simulink model "uav_full_control"  (R2023a)
settings: Solver=FixedStepAuto  StartTime=0.0  StopTime=20  FixedStep=1e-3
undefined symbols (not defined in the file or in its folder): b, c_1, c_2, c_3, c_4, c_5, c_6, c_7, c_8, c_psi, C_SMC, c_z, d, D_rot, D_transl, eps1, eps2, eps3, eps4, eta1, eta2, eta3, eta4, eulerlimit, g, J1, J2, J3, Jr, K, k1, k2, k3, K_lqr, k_phi, K_SMC, k_theta, L, m, Matrix_Force2angular_velocity, R
libraries: simulink x14, control_form_LagrangeSimplified x2, control_form_NL x2, control_form_NL_forces x2, control_form_LagrangeSimplified_forces x1
(part 1 of 2)
settings Model: Creator=Alex  LastModifiedBy=Alex

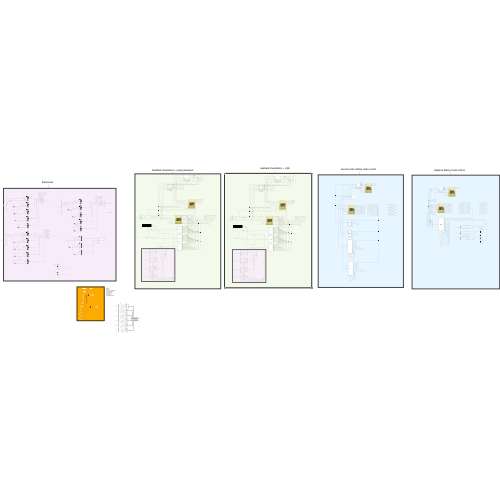
[thumbnail: Simulink's stored preview of the top-level diagram]
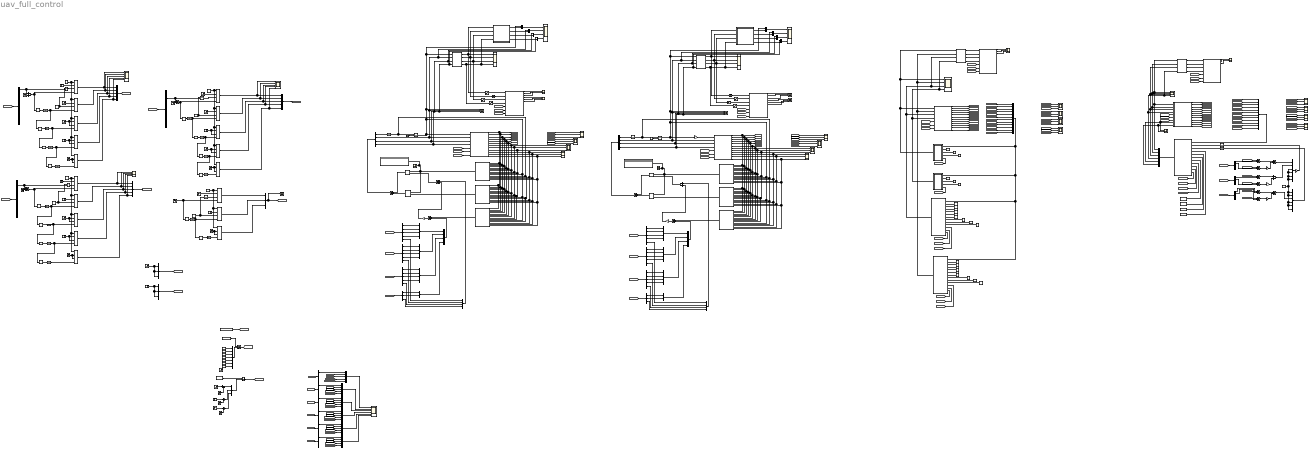
== system uav_full_control ==
  note: enables:
      | - gravity
      | - euler angles saturation
      | - gyroscopic effects
      | - ground effects
      | - drag force
      | - drag torques
      | - wind (translational)
  note: Feedback linearization + LQR
  note: 1 - step
      | 2 - ramp
      | 3 - else
  note: Feedback linearization + pole placement
  note: Adaptive Sliding mode control
  note: Second order sliding mode control
  note: References
  Add{,1,3..4,6..11} (10 alike) : Sum  Inputs=+-
  Add{2,5,12..17} (8 alike) : Sum
  Bus Creator{,1..5} (6 alike) : BusCreator  Inputs=5
  CNL_AngPos{,1..3} (4 alike) : Scope  NumInputPorts=3
  CNL_AngVel{,1..3} (4 alike) : Scope  NumInputPorts=3
  CNL_LinPos{,1..3} (4 alike) : Scope  NumInputPorts=3
  CNL_LinVel{,1..3} (4 alike) : Scope  NumInputPorts=3
  Constant : Constant  Value=K_SMC
  Constant11 : Constant  Value=k_phi
  Constant12 : Constant  Value=k_theta
  Constant13 : Constant  Value=C_SMC
  Constant14 : Constant  Value=0
  Constant15 : Constant  Value=eta1
  Constant16 : Constant  Value=c_z
  Constant17 : Constant  Value=eps3
  Constant20 : Constant  Value=eta3
  Constant21 : Constant  Value=eps4
  Constant22 : Constant  Value=eta4
  Constant23 : Constant  Value=c_5
  Constant24 : Constant  Value=c_6
  Constant25 : Constant  Value=c_7
  Constant26 : Constant  Value=c_8
  Constant29 : Constant  Value=eps1
  Constant3 : Constant  Value=2
  Constant30 : Constant  Value=eta1
  Constant31 : Constant  Value=c_z
  Constant32 : Constant  Value=eps1
  Constant33 : Constant  Value=eta1
  Constant34 : Constant  Value=c_z
  Constant35 : Constant  Value=eps1
  Constant36 : Constant  Value=eta2
  Constant37 : Constant  Value=c_psi
  Constant38 : Constant  Value=eps2
  Constant39 : Constant  Value=c_1
  Constant40 : Constant  Value=c_2
  Constant41 : Constant  Value=c_3
  Constant42 : Constant  Value=c_4
  Constant47 : Constant  Value=[1 0 0 0 1 1 0]
  Constant48 : Constant  Value=[1 1 -5 0 0 0 0 0 0 0 0 0 ]
  Constant49 : Constant  Value=[1 0 0]
  Constant8 : Constant  Value=2
  Demux : Demux
  Demux{1..3,6..8,10..12,14..16} (12 alike) : Demux  Outputs=5
  Demux13 : Demux  Outputs=6
  Demux{4,9,17..19} (5 alike) : Demux  Outputs=3
  Demux20 : Demux  Outputs=12
  Demux21 : Demux  Outputs=12
  Demux22 : Demux  Outputs=12
  Demux5 : Demux
  Discrete Derivative{,1..13} (14 alike) : simulink/Discrete/Discrete Derivative  gainval=1.0  ICPrevScaledInput=0.0  OutMin=[]  OutMax=[]  OutDataType=fixdt(1, 16)  OutScaling=2^-10  DoSatur=off
  Display : Display
  Display1 : Display
  Force2AngularVelocity : Subsystem
  Force2AngularVelocity1 : Subsystem
  Force2AngularVelocity2 : Subsystem
  Force2AngularVelocity3 : Subsystem
  Gain : Gain  Gain=k1
  Gain1 : Gain  Gain=-K_lqr  Multiplication=Matrix(K*u)
  Gain2 : Gain  Gain=-K  Multiplication=Matrix(K*u)
  Gain3 : Gain  Gain=k2
  Gain4 : Gain  Gain=k3
  Gain5 : Gain  Gain=-1
  Gain6 : Gain
  Input_psi : Constant
  Input_x : Constant
  Input_y : Constant
  Input_z : Constant
  Integrator{,2,4..5} (4 alike) : Integrator
  Integrator{1,3,6..7,16} (5 alike) : Integrator  InitialConditionSource=external
  Integrator21 : Integrator  LimitOutput=on  UpperSaturationLimit=pi  LowerSaturationLimit=-pi
  MATLAB Function : MATLAB Function  TreatAsAtomicUnit=on
  MATLAB Function1 : MATLAB Function  TreatAsAtomicUnit=on
  MATLAB Function2 : MATLAB Function  TreatAsAtomicUnit=on
  MATLAB Function3 : MATLAB Function  TreatAsAtomicUnit=on
  MATLAB Function4 : MATLAB Function  TreatAsAtomicUnit=on
  MATLAB Function5 : MATLAB Function  TreatAsAtomicUnit=on
  MATLAB Function6 : MATLAB Function  TreatAsAtomicUnit=on
  Manual Switch : ManualSwitch  CurrentSetting=0
  Manual Switch1 : ManualSwitch  CurrentSetting=0
  Matrix Multiply : Product  Multiplication=Matrix(*)
  Matrix Multiply1 : Product  Multiplication=Matrix(*)
  Multiport Switch{,1..17} (18 alike) : MultiPortSwitch  SaturateOnIntegerOverflow=off  InputSameDT=off
  Mux : Mux  Inputs=5
  Mux1 : Mux  Inputs=5
  Mux{8,10..17,22} (10 alike) : Mux  Inputs=2
  Mux{2,4,6..7,9,18..21,23} (10 alike) : Mux
  Mux24 : Mux  Inputs=12
  Mux25 : Mux  Inputs=6
  Mux26 : Mux  Inputs=6
  Mux{3,27,29,31} (4 alike) : Mux  Inputs=3
  Mux28 : Mux  Inputs=12
  Mux30 : Mux  Inputs=7
  Mux5 : Mux  Inputs=5
  Product : Product  Multiplication=Matrix(*)
  Product1 : Product  Multiplication=Matrix(*)
  STEP0_{1..16} (16 alike) : Step  Time=0  After=0  SampleTime=0
  Saturation{2..5,7..10} (8 alike) : Saturate  UpperLimit=1000  LowerLimit=0
  Scope : Scope
  Scope1 : Scope  NumInputPorts=5
  Scope10 : Scope
  Scope{5,8..9,11,14..17} (8 alike) : Scope  NumInputPorts=4
  Scope{6..7,12..13,18..19} (6 alike) : Scope  NumInputPorts=3
  Scope2 : Scope  NumInputPorts=5
  Scope20 : Scope  NumInputPorts=2
  Scope21 : Scope  NumInputPorts=6
  Scope3 : Scope  NumInputPorts=5
  Scope4 : Scope
  Sine Wave_psi : Sin  SampleTime=0
  Sine Wave_x : Sin  Frequency=0.5  SampleTime=0
  Sine Wave_y : Sin  Frequency=0.5  SampleTime=0
  Sine Wave_z : Sin  Frequency=0.5  SampleTime=0
  Slope_psi : Constant  Value=0.2
  Slope_x : Constant  Value=0.5
  Slope_y : Constant  Value=0.5
  Slope_z : Constant  Value=-1
  Step : Step  Time=25  SampleTime=0
  Step1 : Step  Time=25  SampleTime=0
  Step2 : Step  Time=35  SampleTime=0
  Step3 : Step  Time=50  SampleTime=0
  Step4 : Step  Time=60  SampleTime=0
  Step5 : Step  Time=75  SampleTime=0
  Step6 : Step  Time=85  SampleTime=0
  Step_psi : Step  Time=0  SampleTime=0
  Step_x : Step  Time=0  After=5  SampleTime=0
  Step_y : Step  Time=0  After=5  SampleTime=0
  Step_z : Step  Time=0  After=-7  SampleTime=0
  Subsystem1 : Subsystem
  Subsystem2 : Subsystem
  Sum : Sum  Inputs=|+-
  Sum1 : Sum  Inputs=|+-
  Sum2 : Sum  Inputs=|+-
  Transfer Fcn{,1..13} (14 alike) : TransferFcn  Denominator=[1 1]
  control_form_LagrangeSimplified : control_form_LagrangeSimplified/control_form_LagrangeSimplified  SystemSampleTime=-1  VariantActivationTime=update diagram  Latency=0  AutoFrameSizeCalculation=off
  control_form_LagrangeSimplified1 : control_form_LagrangeSimplified/control_form_LagrangeSimplified  SystemSampleTime=-1  VariantActivationTime=update diagram  Latency=0  AutoFrameSizeCalculation=off
  control_form_LagrangeSimplified_forces : control_form_LagrangeSimplified_forces/control_form_LagrangeSimplified_forces  SystemSampleTime=-1  VariantActivationTime=update diagram  Latency=0  AutoFrameSizeCalculation=off
  control_form_LagrangeSimplified_forces_augumented : Subsystem  AncestorBlock=control_form_LagrangeSimplified_forces/control_form_LagrangeSimplified_forces
  control_form_NL : control_form_NL/control_form_NL  SystemSampleTime=-1  VariantActivationTime=update diagram  Latency=0  AutoFrameSizeCalculation=off
  control_form_NL1 : control_form_NL/control_form_NL  SystemSampleTime=-1  VariantActivationTime=update diagram  Latency=0  AutoFrameSizeCalculation=off
  control_form_NL_forces : control_form_NL_forces/control_form_NL_forces  SystemSampleTime=-1  VariantActivationTime=update diagram  Latency=0  AutoFrameSizeCalculation=off
      settings: LibrarySourceBlock=control_form_NL_forces/control_form_NL
  control_form_NL_forces1 : control_form_NL_forces/control_form_NL_forces  SystemSampleTime=-1  VariantActivationTime=update diagram  Latency=0  AutoFrameSizeCalculation=off
      settings: LibrarySourceBlock=control_form_NL_forces/control_form_NL
  drag force : Constant
  drag torque : Constant
  euler_sat : Constant  Value=0
  gravity : Constant
  ground : Constant  Value=0
  gyro : Constant  Value=0
  u1 : MATLAB Function  TreatAsAtomicUnit=on
  u2 : MATLAB Function  TreatAsAtomicUnit=on
  u3 : MATLAB Function  TreatAsAtomicUnit=on
  u4 : MATLAB Function  TreatAsAtomicUnit=on
  wind : Constant  Value=0
  wires:
  control_form_NL_forces/3 -> MATLAB Function2/3(z), MATLAB Function1/3(z), MATLAB Function/3(z), [CNL_z_LQR]
  control_form_NL_forces/2 -> MATLAB Function2/2(y), MATLAB Function1/2(y), MATLAB Function/2(y), [CNL_y_LQR]
  control_form_NL_forces/1 -> MATLAB Function2/1(x), MATLAB Function1/1(x), MATLAB Function/1(x), [CNL_x_LQR]
  control_form_NL_forces/4 -> MATLAB Function2/4(phi), MATLAB Function1/4(phi), MATLAB Function/4(phi), [CNL_phi_LQR]
  control_form_NL_forces/5 -> MATLAB Function2/5(theta), MATLAB Function1/5(theta), MATLAB Function/5(theta), [CNL_theta_LQR]
  control_form_NL_forces/6 -> MATLAB Function2/6(psi), MATLAB Function1/6(psi), MATLAB Function/6(psi), [CNL_psi_LQR]
  [CNL_x_LQR] -> CNL_LinPos/1
  [CNL_y_LQR] -> CNL_LinPos/2
  [CNL_z_LQR] -> CNL_LinPos/3
  [CNL_phi_LQR] -> CNL_AngPos/1
  [CNL_theta_LQR] -> CNL_AngPos/2
  [CNL_psi_LQR] -> CNL_AngPos/3
  control_form_NL_forces/7 -> MATLAB Function2/7(xdot), MATLAB Function1/7(xdot), MATLAB Function/7(xdot), CNL_LinVel/1
  control_form_NL_forces/8 -> MATLAB Function2/8(ydot), MATLAB Function1/8(ydot), MATLAB Function/8(ydot), CNL_LinVel/2
  control_form_NL_forces/9 -> MATLAB Function/9(zdot), MATLAB Function2/9(zdot), MATLAB Function1/9(zdot), CNL_LinVel/3
  control_form_NL_forces/10 -> CNL_AngVel/1, MATLAB Function2/12(p), MATLAB Function1/12(p), MATLAB Function/12(p)
  control_form_NL_forces/11 -> CNL_AngVel/2, MATLAB Function2/13(q), MATLAB Function1/13(q), MATLAB Function/13(q)
  control_form_NL_forces/12 -> CNL_AngVel/3, MATLAB Function2/14(r), MATLAB Function1/14(r), MATLAB Function/14(r)
  Integrator/1 -> MATLAB Function/11(xi), MATLAB Function2/11(xi), MATLAB Function1/11(xi), Integrator1/1  "xi"
  Product/1 -> Add/2  "alpha"
  MATLAB Function1/1(b) -> Product/2
  MATLAB Function/1(delta_inv) -> Display/1, Scope/1, Matrix Multiply/1, Product/1  "beta"
  Matrix Multiply/1 -> Add/1
  Add1/1 -> Gain1/1  "z"
  Gain1/1 -> Add2/2  "v"
  Add/1 -> Demux/1
  Demux/1 -> Integrator/1  "u1_tilde"
  Integrator1/1 -> Gain6/1, MATLAB Function2/10(zeta), MATLAB Function1/10(zeta), MATLAB Function/10(zeta), Mux10/1, Force2AngularVelocity/1(u1), Scope5/1  "zeta"
  Step_x/1 -> Multiport Switch/2
  Mux/1 -> [xref]
  Constant3/1 -> Integrator1/2
  Mux1/1 -> [yref]
  Step_psi/1 -> Multiport Switch15/2
  Mux3/1 -> [psiref], Scope4/1
  MATLAB Function2/1(transf) -> Add1/1  "z"
  Mux4/1 -> Add1/2
  Input_x/1 -> Multiport Switch4/1, Multiport Switch3/1, Multiport Switch2/1, Multiport Switch1/1, Multiport Switch/1
  STEP0_1/1 -> Multiport Switch1/2
  STEP0_2/1 -> Multiport Switch2/3, Multiport Switch2/2
  STEP0_3/1 -> Multiport Switch3/3, Multiport Switch3/2
  STEP0_4/1 -> Multiport Switch4/3, Multiport Switch4/2
  Multiport Switch/1 -> Scope1/1, Mux/1
  Multiport Switch1/1 -> Scope1/2, Mux/2
  Multiport Switch2/1 -> Scope1/3, Mux/3
  Multiport Switch3/1 -> Scope1/4, Mux/4
  Multiport Switch4/1 -> Scope1/5, Mux/5
  Multiport Switch9/1 -> Scope2/5, Mux1/5
  Multiport Switch8/1 -> Scope2/4, Mux1/4
  Multiport Switch7/1 -> Scope2/3, Mux1/3
  Multiport Switch6/1 -> Scope2/2, Mux1/2
  Multiport Switch5/1 -> Scope2/1, Mux1/1
  STEP0_8/1 -> Multiport Switch9/2, Multiport Switch9/3
  STEP0_7/1 -> Multiport Switch8/2, Multiport Switch8/3
  STEP0_6/1 -> Multiport Switch7/2, Multiport Switch7/3
  STEP0_5/1 -> Multiport Switch6/2
  Input_y/1 -> Multiport Switch5/1, Multiport Switch6/1, Multiport Switch7/1, Multiport Switch8/1, Multiport Switch9/1
  Step_y/1 -> Multiport Switch5/2
  Step_z/1 -> Multiport Switch10/2
  Input_z/1 -> Multiport Switch14/1, Multiport Switch13/1, Multiport Switch12/1, Multiport Switch11/1, Multiport Switch10/1
  STEP0_9/1 -> Multiport Switch11/2
  STEP0_10/1 -> Multiport Switch12/3, Multiport Switch12/2
  STEP0_11/1 -> Multiport Switch13/3, Multiport Switch13/2
  STEP0_12/1 -> Multiport Switch14/3, Multiport Switch14/2
  Multiport Switch10/1 -> Scope3/1, Mux5/1
  Multiport Switch11/1 -> Scope3/2, Mux5/2
  Multiport Switch12/1 -> Scope3/3, Mux5/3
  Multiport Switch13/1 -> Scope3/4, Mux5/4
  Multiport Switch14/1 -> Mux5/5, Scope3/5
  Mux5/1 -> [zref]
  Input_psi/1 -> Multiport Switch17/1, Multiport Switch16/1, Multiport Switch15/1
  STEP0_13/1 -> Multiport Switch16/2
  STEP0_14/1 -> Multiport Switch17/3, Multiport Switch17/2
  Sine Wave_psi/1 -> Discrete Derivative/1, Multiport Switch15/4
  [xref] -> Demux1/1
  Demux1/1 -> Mux2/1
  Demux1/2 -> Mux2/2
  Demux1/3 -> Mux2/3
  Demux1/4 -> Mux2/4
  Mux2/1 -> Mux4/1
  Mux6/1 -> Mux4/2
  Demux2/4 -> Mux6/4
  Demux2/3 -> Mux6/3
  Demux2/2 -> Mux6/2
  Demux2/1 -> Mux6/1
  [yref] -> Demux2/1
  [zref] -> Demux3/1
  Demux3/1 -> Mux7/1
  Demux3/2 -> Mux7/2
  Demux3/3 -> Mux7/3
  Demux3/4 -> Mux7/4
  Mux7/1 -> Mux4/3
  [psiref] -> Demux4/1
  Demux4/1 -> Mux8/1
  Demux4/2 -> Mux8/2
  Mux8/1 -> Mux4/4
  Demux4/3 -> Mux9/4
  Demux3/5 -> Mux9/3
  Demux2/5 -> Mux9/2
  Demux1/5 -> Mux9/1
  Mux9/1 -> Add2/1
  Add2/1 -> Matrix Multiply/2
  control_form_NL/1 -> Scope6/1
  control_form_NL/2 -> Scope6/2
  control_form_NL/3 -> Scope6/3
  control_form_NL/4 -> Scope7/1
  control_form_NL/5 -> Scope7/2
  control_form_NL/6 -> Scope7/3
  Force2AngularVelocity/1(omega_f) -> Subsystem1/1(omega_f), Scope8/1, Saturation2/1  "lqr_front"
  Force2AngularVelocity/2(omega_b) -> Subsystem1/2(omega_b), Scope8/2, Saturation3/1  "lqr_back"
  Force2AngularVelocity/3(omega_l) -> Subsystem1/3(omega_l), Scope8/3, Saturation4/1  "lqr_left"
  Force2AngularVelocity/4(omega_r) -> Saturation5/1, Subsystem1/4(omega_r), Scope8/4  "lqr_right"
  Demux/4 -> control_form_NL_forces/4, Mux13/1, Force2AngularVelocity/4(u4), Scope5/4  "lqr_M3"
  Demux/3 -> control_form_NL_forces/3, Mux12/1, Force2AngularVelocity/3(u3), Scope5/3  "lqr_M2"
  Demux/2 -> control_form_NL_forces/2, Mux11/1, Force2AngularVelocity/2(u2), Scope5/2  "lqr_M1"
  Multiport Switch15/1 -> Mux3/1
  Multiport Switch16/1 -> Mux3/2
  Multiport Switch17/1 -> Mux3/3
  Subsystem1/1(Thrust) -> Mux10/2
  Subsystem1/2(M1) -> Mux11/2
  Subsystem1/3(M2) -> Mux12/2
  Subsystem1/4(M3) -> Mux13/2
  Mux13/1 -> Scope9/4
  Mux12/1 -> Scope9/3
  Mux11/1 -> Scope9/2
  Mux10/1 -> Scope9/1
  Saturation2/1 -> control_form_NL/1
  Saturation3/1 -> control_form_NL/2
  Saturation4/1 -> control_form_NL/3
  Saturation5/1 -> control_form_NL/4
  Mux14/1 -> Scope15/1
  [xref] -> Demux6/1
  Mux16/1 -> Scope15/3
  control_form_NL1/3 -> Scope12/3
  Mux15/1 -> Scope15/2
  Subsystem2/1(Thrust) -> Mux14/2
  Mux17/1 -> Scope15/4
  Demux5/3 -> control_form_NL_forces1/3, Mux16/1, Force2AngularVelocity1/3(u3), Scope11/3  "pp_M2"
  control_form_NL_forces1/4 -> MATLAB Function5/4(phi), MATLAB Function4/4(phi), MATLAB Function3/4(phi), [CNL_phi_PP]
  Subsystem2/2(M1) -> Mux15/2
  Integrator3/1 -> control_form_NL_forces1/1, MATLAB Function5/10(zeta), MATLAB Function4/10(zeta), MATLAB Function3/10(zeta), Mux14/1, Force2AngularVelocity1/1(u1), Scope11/1  "pp_F_thrust"
  Mux23/1 -> Add5/1
  control_form_NL_forces1/5 -> MATLAB Function5/5(theta), MATLAB Function4/5(theta), MATLAB Function3/5(theta), [CNL_theta_PP]
  Demux6/5 -> Mux23/1
  Mux22/1 -> Mux19/4
  Demux7/5 -> Mux23/2
  control_form_NL_forces1/12 -> CNL_AngVel1/3, MATLAB Function5/14(r), MATLAB Function4/14(r), MATLAB Function3/14(r)
  Demux5/4 -> control_form_NL_forces1/4, Mux17/1, Force2AngularVelocity1/4(u4), Scope11/4  "pp_M3"
  Demux6/1 -> Mux18/1
  Demux9/2 -> Mux22/2
  Mux19/1 -> Add4/2
  MATLAB Function4/1(b) -> Product1/2
  Force2AngularVelocity1/4(omega_r) -> Saturation10/1, Subsystem2/4(omega_r), Scope14/4  "pp_right"
  Constant8/1 -> Integrator3/2
  Demux7/2 -> Mux20/2
  Force2AngularVelocity1/3(omega_l) -> Subsystem2/3(omega_l), Scope14/3, Saturation9/1  "pp_left"
  Demux7/3 -> Mux20/3
  control_form_NL1/6 -> Scope13/3
  Demux8/4 -> Mux21/4
  Demux8/5 -> Mux23/3
  Demux9/1 -> Mux22/1
  Mux21/1 -> Mux19/3
  Add5/1 -> Matrix Multiply1/2
  Demux7/1 -> Mux20/1
  Demux9/3 -> Mux23/4
  control_form_NL1/1 -> Scope12/1
  Demux6/3 -> Mux18/3
  control_form_NL1/4 -> Scope13/1
  [yref] -> Demux7/1
  Demux8/2 -> Mux21/2
  Demux8/3 -> Mux21/3
  Demux5/2 -> control_form_NL_forces1/2, Mux15/1, Force2AngularVelocity1/2(u2), Scope11/2  "pp_M1"
  Demux7/4 -> Mux20/4
  control_form_NL1/2 -> Scope12/2
  Demux6/2 -> Mux18/2
  [CNL_y_PP] -> CNL_LinPos1/2
  Mux20/1 -> Mux19/2
  Mux18/1 -> Mux19/1
  Demux6/4 -> Mux18/4
  control_form_NL1/5 -> Scope13/2
  control_form_NL_forces1/9 -> MATLAB Function3/9(zdot), MATLAB Function5/9(zdot), MATLAB Function4/9(zdot), CNL_LinVel1/3
  Force2AngularVelocity1/2(omega_b) -> Subsystem2/2(omega_b), Scope14/2, Saturation8/1  "pp_back"
  Matrix Multiply1/1 -> Add3/1
  MATLAB Function3/1(delta_inv) -> Display1/1, Scope10/1, Matrix Multiply1/1, Product1/1  "beta"
  Demux5/1 -> Integrator2/1  "u1_tilde"
  Add4/1 -> Gain2/1  "z"
  [zref] -> Demux8/1
  MATLAB Function5/1(transf) -> Add4/1  "z"
  control_form_NL_forces1/11 -> CNL_AngVel1/2, MATLAB Function5/13(q), MATLAB Function4/13(q), MATLAB Function3/13(q)
  Subsystem2/3(M2) -> Mux16/2
  Force2AngularVelocity1/1(omega_f) -> Subsystem2/1(omega_f), Scope14/1, Saturation7/1  "pp_front"
  control_form_NL_forces1/8 -> MATLAB Function5/8(ydot), MATLAB Function4/8(ydot), MATLAB Function3/8(ydot), CNL_LinVel1/2
  Gain2/1 -> Add5/2  "v"
  control_form_NL_forces1/2 -> MATLAB Function5/2(y), MATLAB Function4/2(y), MATLAB Function3/2(y), [CNL_y_PP]
  control_form_NL_forces1/3 -> MATLAB Function5/3(z), MATLAB Function4/3(z), MATLAB Function3/3(z), [CNL_z_PP]
  Integrator2/1 -> MATLAB Function3/11(xi), MATLAB Function5/11(xi), MATLAB Function4/11(xi), Integrator3/1  "xi"
  control_form_NL_forces1/7 -> MATLAB Function5/7(xdot), MATLAB Function4/7(xdot), MATLAB Function3/7(xdot), CNL_LinVel1/1
  Product1/1 -> Add3/2  "alpha"
  Subsystem2/4(M3) -> Mux17/2
  Add3/1 -> Demux5/1
  [CNL_phi_PP] -> CNL_AngPos1/1
  Demux8/1 -> Mux21/1
  [CNL_x_PP] -> CNL_LinPos1/1
  [psiref] -> Demux9/1
  [CNL_psi_PP] -> CNL_AngPos1/3
  control_form_NL_forces1/6 -> MATLAB Function5/6(psi), MATLAB Function4/6(psi), MATLAB Function3/6(psi), [CNL_psi_PP]
  control_form_NL_forces1/1 -> MATLAB Function5/1(x), MATLAB Function4/1(x), MATLAB Function3/1(x), [CNL_x_PP]
  [CNL_z_PP] -> CNL_LinPos1/3
  [CNL_theta_PP] -> CNL_AngPos1/2
  control_form_NL_forces1/10 -> CNL_AngVel1/1, MATLAB Function5/12(p), MATLAB Function4/12(p), MATLAB Function3/12(p)
  Saturation7/1 -> control_form_NL1/1
  Saturation8/1 -> control_form_NL1/2
  Saturation9/1 -> control_form_NL1/3
  Saturation10/1 -> control_form_NL1/4
  Add9/1 -> Gain3/1  "ey_dot"
  Add6/1 -> Add12/1  "ex"
  Integrator4/1 -> MATLAB Function6/2(v_hat)
  [CLS_z_ASMC] -> Mux24/3
  Add12/1 -> Mux25/1
  [yref] -> MATLAB Function6/9(yref)
  [CLS_xdot_ASMC] -> Add7/1
  Demux12/2 -> Add7/2
  Demux12/1 -> Add6/2
  Integrator5/1 -> MATLAB Function6/3(fr_hat)
  Demux10/1 -> Add10/2
  [zref] -> Demux10/1
  [psiref] -> MATLAB Function6/11(psiref)
  [xref] -> Demux12/1
  Demux11/1 -> Add8/2
  [CLS_psidot_ASMC] -> CNL_AngVel2/3
  Constant12/1 -> MATLAB Function6/5(k_theta)
  [CLS_psi_ASMC] -> CNL_AngPos2/3
  [CLS_zdot_ASMC] -> CNL_LinVel2/3
  [CLS_psi_ASMC] -> Mux24/6
  [CLS_theta_ASMC] -> Mux24/5
  control_form_LagrangeSimplified_forces_augumented/4(phi) -> [CLS_phi_ASMC]
  [CLS_phi_ASMC] -> Mux24/4
  Constant13/1 -> MATLAB Function6/4(C_SMC)
  [zref] -> MATLAB Function6/10(zref)
  [CLS_z_ASMC] -> CNL_LinPos2/3
  [CLS_zdot_ASMC] -> Mux24/9
  Constant/1 -> MATLAB Function6/7(K_SMC)
  [CLS_psidot_ASMC] -> Mux24/12
  [CLS_phi_ASMC] -> CNL_AngPos2/1
  [CLS_ydot_ASMC] -> Mux24/8
  [CLS_ydot_ASMC] -> CNL_LinVel2/2
  [CLS_y_ASMC] -> Mux24/2
  [CLS_phidot_ASMC] -> Mux24/10
  [CLS_xdot_ASMC] -> Mux24/7
  Mux24/1 -> MATLAB Function6/1(states)
  control_form_LagrangeSimplified_forces_augumented/2(y) -> [CLS_y_ASMC]
  [CLS_thetadot_ASMC] -> Mux24/11
  control_form_LagrangeSimplified_forces_augumented/5(theta) -> [CLS_theta_ASMC]
  control_form_LagrangeSimplified_forces_augumented/6(psi) -> [CLS_psi_ASMC]
  control_form_LagrangeSimplified_forces_augumented/3(z) -> [CLS_z_ASMC]
  control_form_LagrangeSimplified_forces_augumented/10(phidot) -> [CLS_phidot_ASMC]
  control_form_LagrangeSimplified_forces_augumented/7(xdot) -> [CLS_xdot_ASMC]
  [CLS_thetadot_ASMC] -> CNL_AngVel2/2
  [xref] -> MATLAB Function6/8(xref)
  Demux13/2 -> control_form_LagrangeSimplified_forces_augumented/2(M1), Force2AngularVelocity3/2(u2), Scope16/2  "ASMC_M1"
  control_form_LagrangeSimplified_forces_augumented/8(ydot) -> [CLS_ydot_ASMC]
  Demux13/4 -> control_form_LagrangeSimplified_forces_augumented/4(M3), Force2AngularVelocity3/4(u4), Scope16/4  "ASMC_M3"
  Demux13/5 -> Scope20/1, control_form_LagrangeSimplified_forces_augumented/8(u5)
  Demux13/3 -> Scope16/3, Force2AngularVelocity3/3(u3), control_form_LagrangeSimplified_forces_augumented/3(M2)  "ASMC_M2"
  [CLS_x_ASMC] -> CNL_LinPos2/1
  control_form_LagrangeSimplified_forces_augumented/1(x) -> [CLS_x_ASMC]
  control_form_LagrangeSimplified_forces_augumented/11(thetadot) -> [CLS_thetadot_ASMC]
  [CLS_x_ASMC] -> Add6/1
  Add8/1 -> Add13/1  "ey"
  Add10/1 -> Add14/1  "ez"
  Gain4/1 -> Add14/2
  Mux26/1 -> Integrator5/1
  Mux25/1 -> Gain5/1
  [CLS_phidot_ASMC] -> CNL_AngVel2/1
  Gain5/1 -> Integrator4/1
  Add11/1 -> Gain4/1  "ez_dot"
  [CLS_x_ASMC] -> Mux24/1
  [CLS_xdot_ASMC] -> CNL_LinVel2/1
  control_form_LagrangeSimplified_forces_augumented/12(psidot) -> [CLS_psidot_ASMC]
  Add13/1 -> Mux25/2
  Add7/1 -> Gain/1  "ex_dot"
  Demux10/2 -> Add11/2
  Demux11/2 -> Add9/2
  Add14/1 -> Mux26/3
  Demux13/1 -> Force2AngularVelocity3/1(u1), Scope16/1, control_form_LagrangeSimplified_forces_augumented/1(F_thrust)  "ASMC_F_Thrust"
  [CLS_y_ASMC] -> CNL_LinPos2/2
  [CLS_theta_ASMC] -> CNL_AngPos2/2
  [CLS_zdot_ASMC] -> Add11/1
  Constant14/1 -> Mux25/4, Mux25/3, Mux25/5, Mux25/6, Mux26/6, Mux26/5, Mux26/4, Mux26/2, Mux26/1
  Constant11/1 -> MATLAB Function6/6(k_phi)
  control_form_LagrangeSimplified_forces_augumented/9(zdot) -> [CLS_zdot_ASMC]
  Gain3/1 -> Add13/2
  Gain/1 -> Add12/2
  [CLS_z_ASMC] -> Add10/1
  [CLS_y_ASMC] -> Add8/1
  MATLAB Function6/1(u) -> Demux13/1
  [yref] -> Demux11/1
  [CLS_ydot_ASMC] -> Add9/1
  Demux13/6 -> Scope20/2, control_form_LagrangeSimplified_forces_augumented/9(u6)
  Constant32/1 -> u3/9(eps1)
  [thetaref] -> u3/13(thetaref)
  u2/1(u2) -> control_form_LagrangeSimplified_forces/2, Force2AngularVelocity2/2(u2), Scope17/2  "SMC2_M1"
  [CLS_phidot_2SMC] -> CNL_AngVel3/1
  u3/1(u3) -> control_form_LagrangeSimplified_forces/3, Force2AngularVelocity2/3(u3), Scope17/3  "SMC2_M2"
  Constant37/1 -> u4/2(c_psi)
  Constant21/1 -> u2/6(eps4)
  Constant23/1 -> u2/2(c_5)
  Constant34/1 -> u2/8(c_z)
  Constant33/1 -> u2/10(eta1)
  Constant35/1 -> u2/9(eps1)
  control_form_LagrangeSimplified_forces/7 -> [CLS_xdot_2SMC]
  Constant36/1 -> u4/4(eta2)
  Constant31/1 -> u3/8(c_z)
  control_form_LagrangeSimplified_forces/4 -> [CLS_phi_2SMC]
  Constant30/1 -> u3/10(eta1)
  u4/1(u4) -> control_form_LagrangeSimplified_forces/4, Force2AngularVelocity2/4(u4), Scope17/4  "SMC2_M3"
  Constant25/1 -> u2/4(c_7)
  [CLS_zdot_2SMC] -> CNL_LinVel3/3
  Constant42/1 -> u3/5(c_4)
  [CLS_x_2SMC] -> Mux28/1
  control_form_LagrangeSimplified_forces/11 -> [CLS_thetadot_2SMC]
  Constant22/1 -> u2/7(eta4)
  Constant39/1 -> u3/2(c_1)
  Constant26/1 -> u2/5(c_8)
  [CLS_z_2SMC] -> Mux28/3
  Constant24/1 -> u2/3(c_6)
  Constant16/1 -> u1/2(c_z)
  [yref] -> u2/12(yref)
  Constant41/1 -> u3/4(c_3)
  [CLS_psidot_2SMC] -> Mux28/12
  [CLS_xdot_2SMC] -> CNL_LinVel3/1
  [CLS_y_2SMC] -> CNL_LinPos3/2
  [zref] -> u1/5(zref)
  Constant38/1 -> u4/3(eps2)
  [CLS_thetadot_2SMC] -> CNL_AngVel3/2
  [zref] -> u3/11(zref)
  [zref] -> u2/11(zref)
  [xref] -> u3/12(xref)
  Mux28/1 -> u2/1(states), u3/1(states), u4/1(states), u1/1(states)
  Constant20/1 -> u3/7(eta3)
  [CLS_theta_2SMC] -> CNL_AngPos3/2
  [CLS_phidot_2SMC] -> Mux28/10
  Constant29/1 -> u1/3(eps1)
  [CLS_psi_2SMC] -> CNL_AngPos3/3
  control_form_LagrangeSimplified_forces/12 -> [CLS_psidot_2SMC]
  [CLS_ydot_2SMC] -> Mux28/8
  [CLS_theta_2SMC] -> Mux28/5
  control_form_LagrangeSimplified_forces/6 -> [CLS_psi_2SMC]
  [phiref] -> u2/13(phiref)
  [psiref] -> u4/5(psiref)
  [CLS_z_2SMC] -> CNL_LinPos3/3
  [CLS_zdot_2SMC] -> Mux28/9
  control_form_LagrangeSimplified_forces/5 -> [CLS_theta_2SMC]
  u1/1(u1) -> control_form_LagrangeSimplified_forces/1, Scope17/1, Force2AngularVelocity2/1(u1)  "SMC2_F_Thrust"
  control_form_LagrangeSimplified_forces/10 -> [CLS_phidot_2SMC]
  [CLS_thetadot_2SMC] -> Mux28/11
  [CLS_phi_2SMC] -> CNL_AngPos3/1
  control_form_LagrangeSimplified_forces/9 -> [CLS_zdot_2SMC]
  [CLS_psi_2SMC] -> Mux28/6
  Constant15/1 -> u1/4(eta1)
  [CLS_y_2SMC] -> Mux28/2
  control_form_LagrangeSimplified_forces/3 -> [CLS_z_2SMC]
  control_form_LagrangeSimplified_forces/2 -> [CLS_y_2SMC]
  [CLS_phi_2SMC] -> Mux28/4
  Constant17/1 -> u3/6(eps3)
  [CLS_ydot_2SMC] -> CNL_LinVel3/2
  [CLS_psidot_2SMC] -> CNL_AngVel3/3
  Constant40/1 -> u3/3(c_2)
  control_form_LagrangeSimplified_forces/8 -> [CLS_ydot_2SMC]
  [CLS_xdot_2SMC] -> Mux28/7
  control_form_LagrangeSimplified_forces/1 -> [CLS_x_2SMC]
  [CLS_x_2SMC] -> CNL_LinPos3/1
  Mux29/1 -> [phiref]
  STEP0_16/1 -> Mux29/1, Mux29/2, Mux29/3
  STEP0_15/1 -> Mux27/2, Mux27/3, Mux27/1
  Mux27/1 -> [thetaref]
  Force2AngularVelocity2/1(omega_f) -> control_form_LagrangeSimplified1/1  "SMC2_front"
  Force2AngularVelocity2/2(omega_b) -> control_form_LagrangeSimplified1/2  "SMC2_back"
  Force2AngularVelocity2/3(omega_l) -> control_form_LagrangeSimplified1/3  "SMC2_left"
  Force2AngularVelocity2/4(omega_r) -> control_form_LagrangeSimplified1/4  "SMC2_right"
  Force2AngularVelocity3/1(omega_f) -> control_form_LagrangeSimplified/1  "ASMC_front"
  Force2AngularVelocity3/2(omega_b) -> control_form_LagrangeSimplified/2  "ASMC_back"
  Force2AngularVelocity3/3(omega_l) -> control_form_LagrangeSimplified/3  "ASMC_left"
  Force2AngularVelocity3/4(omega_r) -> control_form_LagrangeSimplified/4  "ASMC_right"
  control_form_LagrangeSimplified1/1 -> Scope18/1
  control_form_LagrangeSimplified1/2 -> Scope18/2
  control_form_LagrangeSimplified1/3 -> Scope18/3
  control_form_LagrangeSimplified/1 -> Scope19/1
  control_form_LagrangeSimplified/2 -> Scope19/2
  control_form_LagrangeSimplified/3 -> Scope19/3
  Constant48/1 -> [initial_values]
  Manual Switch/1 -> [enables]
  Constant49/1 -> Manual Switch1/1
  [initial_values] -> control_form_NL1/5
  [enables] -> control_form_NL1/6
  [wind_power] -> control_form_NL1/7
  [initial_values] -> control_form_NL_forces1/5
  [enables] -> control_form_NL_forces1/6
  [wind_power] -> control_form_NL_forces1/7
  [initial_values] -> control_form_NL_forces/5
  [enables] -> control_form_NL_forces/6
  [wind_power] -> control_form_NL_forces/7
  [initial_values] -> control_form_NL/5
  [enables] -> control_form_NL/6
  [wind_power] -> control_form_NL/7
  [initial_values] -> control_form_LagrangeSimplified_forces/5
  [enables] -> control_form_LagrangeSimplified_forces/6
  [wind_power] -> control_form_LagrangeSimplified_forces/7
  [initial_values] -> control_form_LagrangeSimplified1/5
  [enables] -> control_form_LagrangeSimplified1/6
  [wind_power] -> control_form_LagrangeSimplified1/7
  [initial_values] -> control_form_LagrangeSimplified_forces_augumented/5(initial_value)
  [enables] -> control_form_LagrangeSimplified_forces_augumented/6(enables)
  [wind_power] -> control_form_LagrangeSimplified_forces_augumented/7(wind_power)
  [initial_values] -> control_form_LagrangeSimplified/5
  [enables] -> control_form_LagrangeSimplified/6
  [wind_power] -> control_form_LagrangeSimplified/7
  Bus Creator/1 -> Scope21/1  "x"
  Bus Creator1/1 -> Scope21/2  "y"
  Bus Creator2/1 -> Scope21/3  "z"
  Bus Creator3/1 -> Scope21/4  "phi"
  Bus Creator4/1 -> Scope21/5  "theta"
  Bus Creator5/1 -> Scope21/6  "psi"
  [CNL_x_PP] -> Bus Creator/2  "x_pp"
  [CNL_y_PP] -> Bus Creator1/2  "y_pp"
  [CNL_z_PP] -> Bus Creator2/2  "z_pp"
  [CNL_phi_PP] -> Bus Creator3/2  "phi_pp"
  [CNL_theta_PP] -> Bus Creator4/2  "theta_pp"
  [CNL_psi_PP] -> Bus Creator5/2  "psi_pp"
  [xref] -> Demux14/1
  Demux14/1 -> Bus Creator/1  "xref"
  [yref] -> Demux15/1
  Demux15/1 -> Bus Creator1/1  "yref"
  Demux16/1 -> Bus Creator2/1  "zref"
  [zref] -> Demux16/1
  Demux17/1 -> Bus Creator3/1  "phiref"
  [phiref] -> Demux17/1
  Demux18/1 -> Bus Creator4/1  "thetaref"
  [thetaref] -> Demux18/1
  Demux19/1 -> Bus Creator5/1  "psiref"
  [psiref] -> Demux19/1
  [CNL_psi_LQR] -> Bus Creator5/3  "psi_lqr"
  [CLS_psi_2SMC] -> Bus Creator5/4  "psi_2smc"
  [CLS_psi_ASMC] -> Bus Creator5/5  "psi_asmc"
  [CNL_theta_LQR] -> Bus Creator4/3  "theta_lqr"
  [CNL_x_LQR] -> Bus Creator/3  "x_lqr"
  [CNL_y_LQR] -> Bus Creator1/3  "y_lqr"
  [CNL_z_LQR] -> Bus Creator2/3  "z_lqr"
  [CNL_phi_LQR] -> Bus Creator3/3  "phi_lqr"
  [CLS_x_2SMC] -> Bus Creator/4  "x_2smc"
  [CLS_y_2SMC] -> Bus Creator1/4  "y_2smc"
  [CLS_z_2SMC] -> Bus Creator2/4  "z_2smc"
  [CLS_phi_2SMC] -> Bus Creator3/4  "phi_2smc"
  [CLS_theta_2SMC] -> Bus Creator4/4  "theta_2smc"
  [CLS_x_ASMC] -> Bus Creator/5  "x_asmc"
  [CLS_y_ASMC] -> Bus Creator1/5  "y_asmc"
  [CLS_z_ASMC] -> Bus Creator2/5  "z_asmc"
  [CLS_phi_ASMC] -> Bus Creator3/5  "phi_asmc"
  [CLS_theta_ASMC] -> Bus Creator4/5  "theta_asmc"
  Slope_x/1 -> Integrator6/1, Multiport Switch1/3
  Integrator6/1 -> Multiport Switch/3
  Slope_y/1 -> Integrator7/1, Multiport Switch6/3
  Integrator7/1 -> Multiport Switch5/3
  Demux20/2 -> Integrator7/2, Add16/1
  [initial_values] -> Demux20/1
  [initial_values] -> Demux21/1
  Demux21/1 -> Add15/1, Integrator6/2
  [initial_values] -> Demux22/1
  Slope_z/1 -> Integrator16/1, Multiport Switch11/3
  Integrator16/1 -> Multiport Switch10/3
  Demux22/3 -> Add17/1, Integrator16/2
  Integrator21/1 -> Multiport Switch15/3
  Slope_psi/1 -> Integrator21/1, Multiport Switch16/3
  Discrete Derivative/1 -> Transfer Fcn1/1
  Discrete Derivative1/1 -> Transfer Fcn/1
  Transfer Fcn/1 -> Multiport Switch17/4
  Transfer Fcn1/1 -> Discrete Derivative1/1, Multiport Switch16/4
  Add17/1 -> Multiport Switch10/4, Discrete Derivative2/1
  Discrete Derivative2/1 -> Transfer Fcn2/1
  Transfer Fcn2/1 -> Multiport Switch11/4, Discrete Derivative3/1
  Discrete Derivative3/1 -> Transfer Fcn3/1
  Transfer Fcn3/1 -> Discrete Derivative4/1, Multiport Switch12/4
  Discrete Derivative4/1 -> Transfer Fcn4/1
  Transfer Fcn4/1 -> Discrete Derivative5/1, Multiport Switch13/4
  Discrete Derivative5/1 -> Transfer Fcn5/1
  Transfer Fcn5/1 -> Multiport Switch14/4
  Discrete Derivative6/1 -> Transfer Fcn6/1
  Add16/1 -> Multiport Switch5/4, Discrete Derivative6/1
  Transfer Fcn6/1 -> Discrete Derivative7/1, Multiport Switch6/4
  Discrete Derivative7/1 -> Transfer Fcn7/1
  Transfer Fcn7/1 -> Discrete Derivative8/1, Multiport Switch7/4
  Discrete Derivative8/1 -> Transfer Fcn8/1
  Transfer Fcn8/1 -> Discrete Derivative9/1, Multiport Switch8/4
  Discrete Derivative9/1 -> Transfer Fcn9/1
  Transfer Fcn9/1 -> Multiport Switch9/4
  Discrete Derivative10/1 -> Transfer Fcn10/1
  Add15/1 -> Multiport Switch/4, Discrete Derivative10/1
  Transfer Fcn10/1 -> Discrete Derivative11/1, Multiport Switch1/4
  Discrete Derivative11/1 -> Transfer Fcn11/1
  Transfer Fcn11/1 -> Discrete Derivative12/1, Multiport Switch2/4
  Discrete Derivative12/1 -> Transfer Fcn12/1
  Transfer Fcn12/1 -> Discrete Derivative13/1, Multiport Switch3/4
  Discrete Derivative13/1 -> Transfer Fcn13/1
  Transfer Fcn13/1 -> Multiport Switch4/4
  Sine Wave_x/1 -> Add15/2
  Sine Wave_y/1 -> Add16/2
  Sine Wave_z/1 -> Add17/2
  Gain6/1 -> control_form_NL_forces/1  "lqr_F_thrust"
  Mux30/1 -> Manual Switch/2
  Constant47/1 -> Manual Switch/1
  gravity/1 -> Mux30/1
  euler_sat/1 -> Mux30/2
  gyro/1 -> Mux30/3
  ground/1 -> Mux30/4
  drag force/1 -> Mux30/5
  drag torque/1 -> Mux30/6
  wind/1 -> Mux30/7
  Mux31/1 -> Manual Switch1/2
  Manual Switch1/1 -> [wind_power]
  Step1/1 -> Sum/1
  Sum/1 -> Mux31/1
  Step2/1 -> Sum/2
  Step3/1 -> Sum1/1
  Step4/1 -> Sum1/2
  Sum1/1 -> Mux31/2
  Step5/1 -> Sum2/1
  Step6/1 -> Sum2/2
  Sum2/1 -> Mux31/3

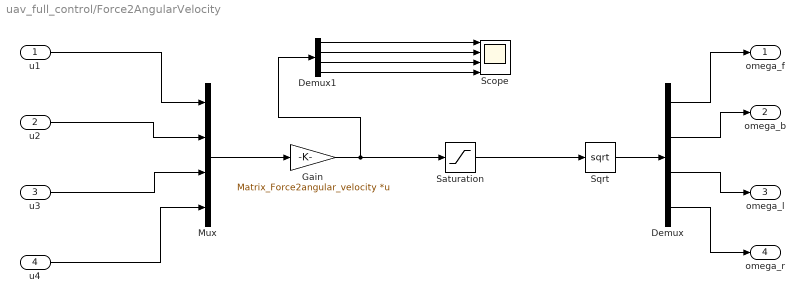
== system uav_full_control/Force2AngularVelocity ==
  u1 : Inport
  u2 : Inport  Port=2
  u3 : Inport  Port=3
  u4 : Inport  Port=4
  Demux : Demux
  Demux1 : Demux
  Gain : Gain  Gain=Matrix_Force2angular_velocity  Multiplication=Matrix(K*u)
  Mux : Mux
  Saturation : Saturate  UpperLimit=inf  LowerLimit=0
  Scope : Scope  NumInputPorts=4
  Sqrt : Sqrt
  omega_f : Outport
  omega_b : Outport  Port=2
  omega_l : Outport  Port=3
  omega_r : Outport  Port=4
  wires:
  u3/1 -> Mux/3
  u2/1 -> Mux/2
  u4/1 -> Mux/4
  u1/1 -> Mux/1
  Mux/1 -> Gain/1
  Sqrt/1 -> Demux/1
  Demux/3 -> omega_l/1
  Demux/2 -> omega_b/1
  Demux/4 -> omega_r/1
  Demux/1 -> omega_f/1
  Demux1/1 -> Scope/1
  Demux1/2 -> Scope/2
  Demux1/3 -> Scope/3
  Demux1/4 -> Scope/4
  Gain/1 -> Saturation/1, Demux1/1
  Saturation/1 -> Sqrt/1

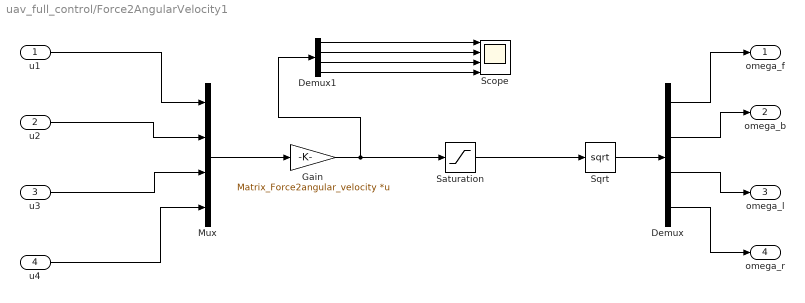
== system uav_full_control/Force2AngularVelocity1 ==
  u1 : Inport
  u2 : Inport  Port=2
  u3 : Inport  Port=3
  u4 : Inport  Port=4
  Demux : Demux
  Demux1 : Demux
  Gain : Gain  Gain=Matrix_Force2angular_velocity  Multiplication=Matrix(K*u)
  Mux : Mux
  Saturation : Saturate  UpperLimit=inf  LowerLimit=0
  Scope : Scope  NumInputPorts=4
  Sqrt : Sqrt
  omega_f : Outport
  omega_b : Outport  Port=2
  omega_l : Outport  Port=3
  omega_r : Outport  Port=4
  wires:
  u3/1 -> Mux/3
  u2/1 -> Mux/2
  u4/1 -> Mux/4
  u1/1 -> Mux/1
  Mux/1 -> Gain/1
  Sqrt/1 -> Demux/1
  Demux/3 -> omega_l/1
  Demux/2 -> omega_b/1
  Demux/4 -> omega_r/1
  Demux/1 -> omega_f/1
  Demux1/1 -> Scope/1
  Demux1/2 -> Scope/2
  Demux1/3 -> Scope/3
  Demux1/4 -> Scope/4
  Gain/1 -> Saturation/1, Demux1/1
  Saturation/1 -> Sqrt/1

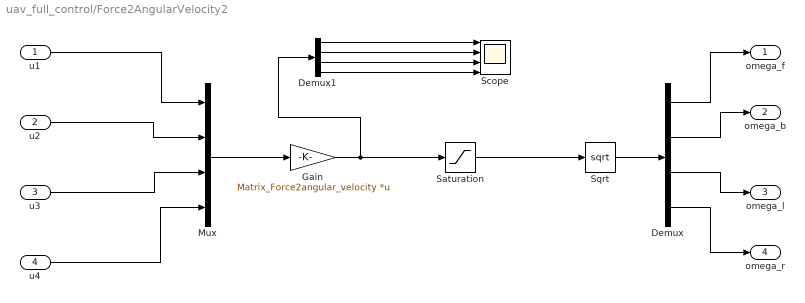
== system uav_full_control/Force2AngularVelocity2 ==
  u1 : Inport
  u2 : Inport  Port=2
  u3 : Inport  Port=3
  u4 : Inport  Port=4
  Demux : Demux
  Demux1 : Demux
  Gain : Gain  Gain=Matrix_Force2angular_velocity  Multiplication=Matrix(K*u)
  Mux : Mux
  Saturation : Saturate  UpperLimit=inf  LowerLimit=0
  Scope : Scope  NumInputPorts=4
  Sqrt : Sqrt
  omega_f : Outport
  omega_b : Outport  Port=2
  omega_l : Outport  Port=3
  omega_r : Outport  Port=4
  wires:
  Saturation/1 -> Sqrt/1
  Gain/1 -> Demux1/1, Saturation/1
  Demux1/4 -> Scope/4
  Demux1/3 -> Scope/3
  Demux1/2 -> Scope/2
  Demux1/1 -> Scope/1
  Demux/1 -> omega_f/1
  Demux/4 -> omega_r/1
  Demux/2 -> omega_b/1
  Demux/3 -> omega_l/1
  Sqrt/1 -> Demux/1
  Mux/1 -> Gain/1
  u1/1 -> Mux/1
  u4/1 -> Mux/4
  u2/1 -> Mux/2
  u3/1 -> Mux/3

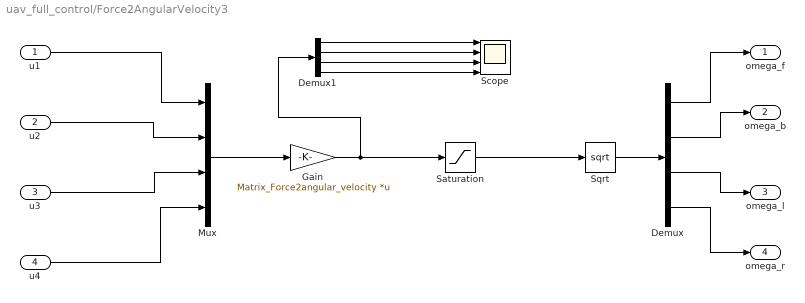
== system uav_full_control/Force2AngularVelocity3 ==
  u1 : Inport
  u2 : Inport  Port=2
  u3 : Inport  Port=3
  u4 : Inport  Port=4
  Demux : Demux
  Demux1 : Demux
  Gain : Gain  Gain=Matrix_Force2angular_velocity  Multiplication=Matrix(K*u)
  Mux : Mux
  Saturation : Saturate  UpperLimit=inf  LowerLimit=0
  Scope : Scope  NumInputPorts=4
  Sqrt : Sqrt
  omega_f : Outport
  omega_b : Outport  Port=2
  omega_l : Outport  Port=3
  omega_r : Outport  Port=4
  wires:
  u3/1 -> Mux/3
  u2/1 -> Mux/2
  u4/1 -> Mux/4
  u1/1 -> Mux/1
  Mux/1 -> Gain/1
  Sqrt/1 -> Demux/1
  Demux/3 -> omega_l/1
  Demux/2 -> omega_b/1
  Demux/4 -> omega_r/1
  Demux/1 -> omega_f/1
  Demux1/1 -> Scope/1
  Demux1/2 -> Scope/2
  Demux1/3 -> Scope/3
  Demux1/4 -> Scope/4
  Gain/1 -> Saturation/1, Demux1/1
  Saturation/1 -> Sqrt/1

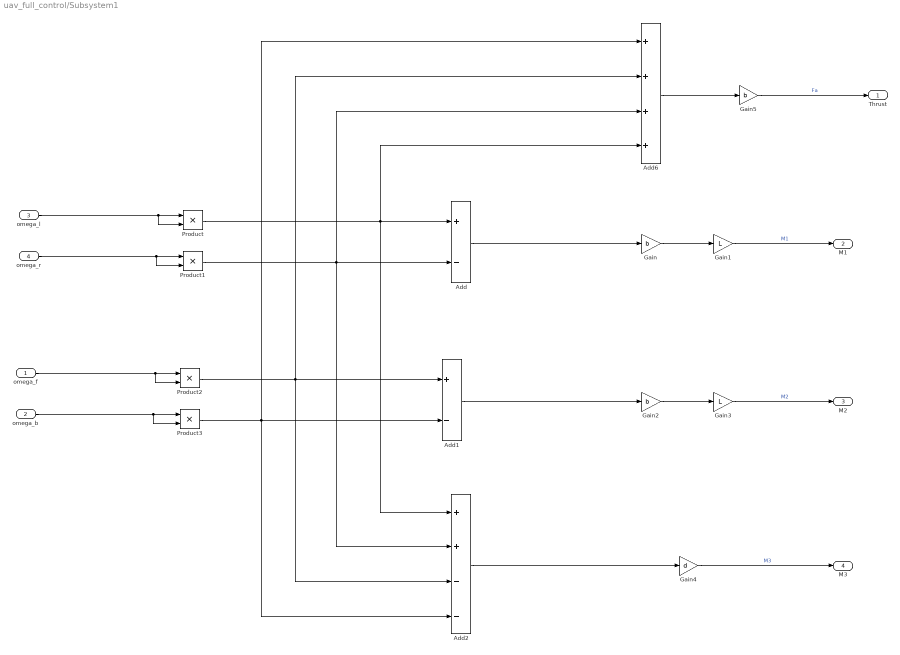
== system uav_full_control/Subsystem1 ==
  omega_f : Inport
  omega_b : Inport  Port=2
  omega_l : Inport  Port=3
  omega_r : Inport  Port=4
  Add : Sum  Inputs=+-
  Add1 : Sum  Inputs=+-
  Add2 : Sum  Inputs=++--
  Add6 : Sum  Inputs=++++
  Gain : Gain  Gain=b
  Gain1 : Gain  Gain=L
  Gain2 : Gain  Gain=b
  Gain3 : Gain  Gain=L
  Gain4 : Gain  Gain=d
  Gain5 : Gain  Gain=b
  Product{,1..3} (4 alike) : Product
  Thrust : Outport
  M1 : Outport  Port=2
  M2 : Outport  Port=3
  M3 : Outport  Port=4
  wires:
  Add/1 -> Gain/1
  Gain2/1 -> Gain3/1
  omega_b/1 -> Product3/1, Product3/2
  Product3/1 -> Add6/1, Add2/4, Add1/2
  Product/1 -> Add6/4, Add2/1, Add/1
  omega_f/1 -> Product2/1, Product2/2
  omega_r/1 -> Product1/1, Product1/2
  Add1/1 -> Gain2/1
  Gain4/1 -> M3/1  "M3"
  Add2/1 -> Gain4/1
  Product1/1 -> Add6/3, Add2/2, Add/2
  omega_l/1 -> Product/1, Product/2
  Gain3/1 -> M2/1  "M2"
  Product2/1 -> Add6/2, Add2/3, Add1/1
  Gain/1 -> Gain1/1
  Gain1/1 -> M1/1  "M1"
  Add6/1 -> Gain5/1
  Gain5/1 -> Thrust/1  "Fa"

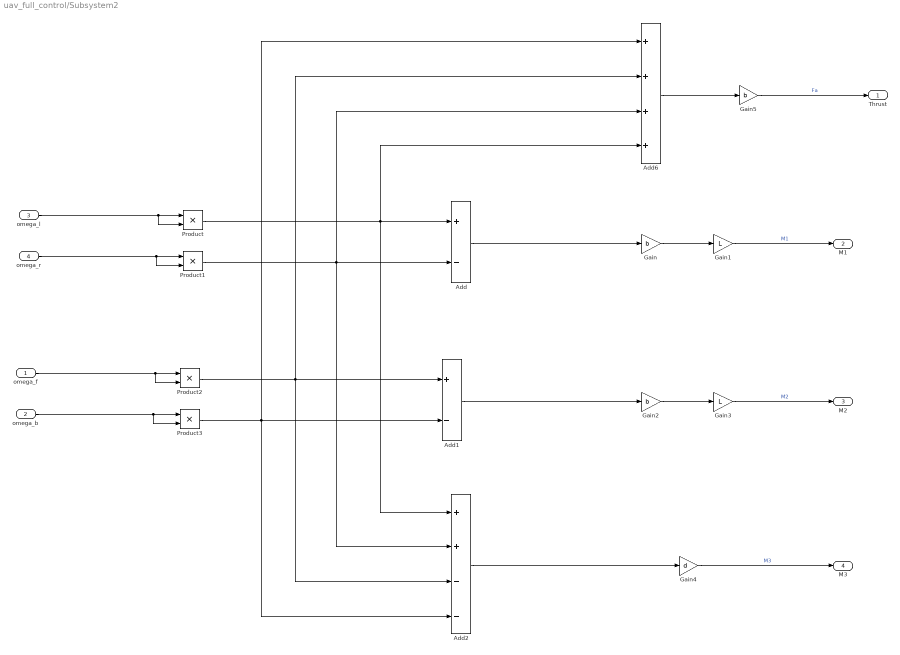
== system uav_full_control/Subsystem2 ==
  omega_f : Inport
  omega_b : Inport  Port=2
  omega_l : Inport  Port=3
  omega_r : Inport  Port=4
  Add : Sum  Inputs=+-
  Add1 : Sum  Inputs=+-
  Add2 : Sum  Inputs=++--
  Add6 : Sum  Inputs=++++
  Gain : Gain  Gain=b
  Gain1 : Gain  Gain=L
  Gain2 : Gain  Gain=b
  Gain3 : Gain  Gain=L
  Gain4 : Gain  Gain=d
  Gain5 : Gain  Gain=b
  Product{,1..3} (4 alike) : Product
  Thrust : Outport
  M1 : Outport  Port=2
  M2 : Outport  Port=3
  M3 : Outport  Port=4
  wires:
  Add/1 -> Gain/1
  Gain2/1 -> Gain3/1
  omega_b/1 -> Product3/1, Product3/2
  Product3/1 -> Add6/1, Add2/4, Add1/2
  Product/1 -> Add6/4, Add2/1, Add/1
  omega_f/1 -> Product2/1, Product2/2
  omega_r/1 -> Product1/1, Product1/2
  Add1/1 -> Gain2/1
  Gain4/1 -> M3/1  "M3"
  Add2/1 -> Gain4/1
  Product1/1 -> Add6/3, Add2/2, Add/2
  omega_l/1 -> Product/1, Product/2
  Gain3/1 -> M2/1  "M2"
  Product2/1 -> Add6/2, Add2/3, Add1/1
  Gain/1 -> Gain1/1
  Gain1/1 -> M1/1  "M1"
  Add6/1 -> Gain5/1
  Gain5/1 -> Thrust/1  "Fa"

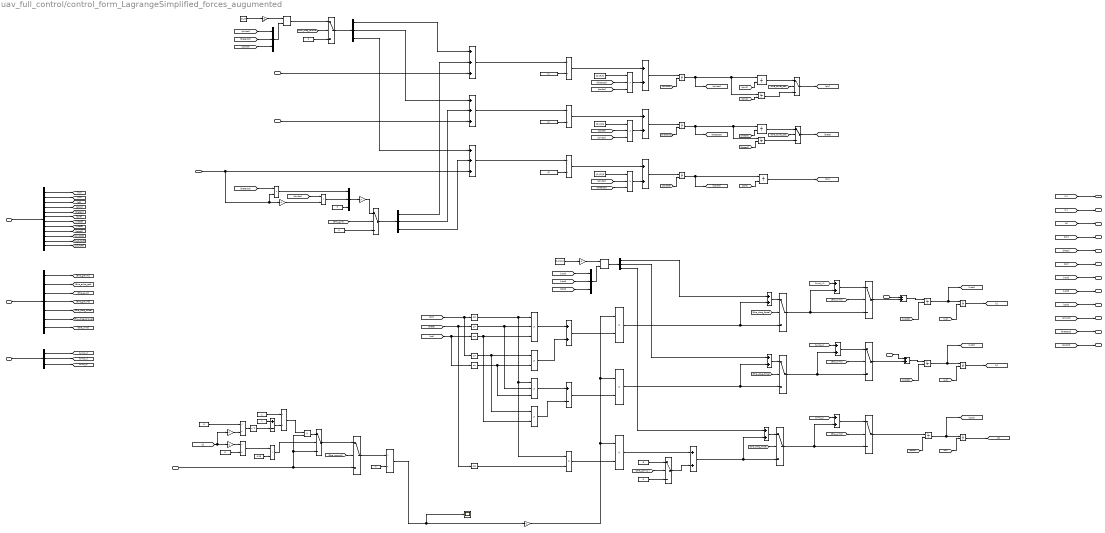
== system uav_full_control/control_form_LagrangeSimplified_forces_augumented ==
  note: Drag force
  note: Translational dynamics
  note: Simplified Euler equations of motion
      | Rotational dynamics
  note: Gyro
  note: Drag torque
  note: Ground
  F_thrust : Inport
  M1 : Inport  Port=2
  M2 : Inport  Port=3
  M3 : Inport  Port=4
  initial_value : Inport  Port=5
  enables : Inport  Port=6
  wind_power : Inport  Port=7
  u5 : Inport  Port=8
  u6 : Inport  Port=9
  Add{,1,3..5,18,20..24,33..34} (13 alike) : Sum
  Add10 : Sum  Inputs=+++
  Add11 : Sum  Inputs=+++
  Add19 : Sum  Inputs=+-
  Add25 : Sum  Inputs=+++
  Add26 : Sum  Inputs=+-
  Constant : Constant  Value=J1
  Constant1 : Constant  Value=J2
  Constant10 : Constant  Value=R
  Constant{9,11,13,20} (4 alike) : Constant  Value=0
  Constant12 : Constant  Value=D_rot
  Constant14 : Constant  Value=0.25
  Constant15 : Constant  Value=R
  Constant16 : Constant
  Constant17 : Constant
  Constant19 : Constant  Value=D_transl
  Constant2 : Constant  Value=J3
  Constant21 : Constant  Value=g
  Constant3 : Constant  Value=(J2-J3)/J1
  Constant4 : Constant  Value=(J3-J1)/J2
  Constant5 : Constant  Value=(J1-J2)/J3
  Constant6 : Constant  Value=m
  Cos : Trigonometry  Operator=cos
  Cos1 : Trigonometry  Operator=cos
  Demux : Demux  Outputs=12
  Demux1 : Demux  Outputs=7
  Demux{2..3,5..6} (4 alike) : Demux  Outputs=3
  Divide{,1..2,5..8} (7 alike) : Product  Inputs=*/
  Gain10 : Gain  Gain=4
  Gain{6,8..9,12..13} (5 alike) : Gain  Gain=-1
  Gain7 : Gain  Gain=Jr
  Integrator{,1..3,7..11,13..14} (11 alike) : Integrator  InitialConditionSource=external
  Integrator4 : Integrator  InitialConditionSource=external  LimitOutput=on  UpperSaturationLimit=eulerlimit  LowerSaturationLimit=-eulerlimit
  Integrator5 : Integrator  InitialConditionSource=external  LimitOutput=on  UpperSaturationLimit=eulerlimit  LowerSaturationLimit=-eulerlimit
  Integrator6 : Integrator  InitialConditionSource=external  LimitOutput=on  UpperSaturationLimit=pi  LowerSaturationLimit=-pi
  Mux : Mux  Inputs=3
  Mux1 : Mux  Inputs=3
  Mux3 : Mux  Inputs=3
  Product16 : Product  Multiplication=Matrix(*)
  Product{17..19,28,30..34} (9 alike) : Product
  Product{4..6,27,29} (5 alike) : Product  Inputs=3
  Product35 : Product  Multiplication=Matrix(*)
  Relational Operator : RelationalOperator  Operator=>  OutDataTypeStr=boolean  RndMeth=Simplest  InputSameDT=off
  Scope1 : Scope
  Sin12 : Trigonometry
  Sin13 : Trigonometry  Operator=cos
  Sin14 : Trigonometry
  Sin15 : Trigonometry
  Square : Math  Operator=square
  Switch{,1..5,11..17} (13 alike) : Switch  Criteria=u2 ~= 0  SaturateOnIntegerOverflow=off  InputSameDT=off
  x : Outport
  y : Outport  Port=2
  z : Outport  Port=3
  phi : Outport  Port=4
  theta : Outport  Port=5
  psi : Outport  Port=6
  xdot : Outport  Port=7
  ydot : Outport  Port=8
  zdot : Outport  Port=9
  phidot : Outport  Port=10
  thetadot : Outport  Port=11
  psidot : Outport  Port=12
  wires:
  [Ena_drag_force] -> Switch13/2
  Add20/1 -> Add21/2, Switch13/3
  Add21/1 -> Switch13/1
  Mux3/1 -> Product35/2
  [zdot] -> Mux3/3
  [xdot] -> Mux3/1
  Gain13/1 -> Product35/1
  Constant19/1 -> Gain13/1
  [ydot] -> Mux3/2
  Add22/1 -> Switch14/1
  Product33/1 -> Switch14/3, Add22/2
  [Ena_drag_force] -> Switch14/2
  [Ena_drag_force] -> Switch15/2
  Product32/1 -> Switch15/3, Add23/2
  Add23/1 -> Switch15/1
  Product35/1 -> Demux6/1
  Demux6/2 -> Add22/1
  Demux6/3 -> Add21/1
  Switch13/1 -> Add34/2, Switch16/3
  Switch14/1 -> Add33/2, Switch17/3
  Switch15/1 -> Add24/2, Switch12/3
  [Ena_wind] -> Switch17/2
  [Ena_wind] -> Switch16/2
  [Ena_wind] -> Switch12/2
  Add24/1 -> Switch12/1
  Add33/1 -> Switch17/1
  Add34/1 -> Switch16/1
  [wind_x] -> Add24/1
  [wind_y] -> Add33/1
  [wind_z] -> Add34/1
  Demux6/1 -> Add23/1
  Switch11/1 -> Add20/2  "gravity"
  [Ena_gravity] -> Switch11/2
  Constant21/1 -> Switch11/1
  Constant20/1 -> Switch11/3
  Gain12/1 -> Product34/1, Product33/1, Product32/1
  Cos1/1 -> Product30/2, Product27/3
  Product27/1 -> Add18/1
  [x0] -> Integrator14/2
  Integrator13/1 -> [y]
  [theta] -> Sin13/1, Sin14/1
  Add18/1 -> Product32/2
  [psi] -> Cos1/1, Sin12/1
  Product31/1 -> Product34/2
  Integrator11/1 -> [z]
  Integrator10/1 -> Integrator11/1, [zdot]
  Product34/1 -> Add20/1
  [zdot0] -> Integrator10/2
  [xdot0] -> Integrator3/2
  Product28/1 -> Add18/2
  Add19/1 -> Product33/2
  Integrator3/1 -> Integrator14/1, [xdot]
  Sin13/1 -> Product31/2
  [y0] -> Integrator13/2
  Integrator14/1 -> [x]
  [ydot0] -> Integrator9/2
  Product29/1 -> Add19/1
  Cos/1 -> Product31/1, Product29/1, Product27/1
  Sin14/1 -> Product29/2, Product27/2
  [phi] -> Sin15/1, Cos/1
  Switch16/1 -> Integrator10/1
  Switch17/1 -> Add1/2
  Integrator9/1 -> Integrator13/1, [ydot]
  Sin12/1 -> Product29/3, Product28/2
  Sin15/1 -> Product30/1, Product28/1
  [z0] -> Integrator11/2
  Product30/1 -> Add19/2
  Switch12/1 -> Add/2
  Demux5/3 -> [wind_z]
  Demux5/2 -> [wind_y]
  Demux5/1 -> [wind_x]
  Demux2/3 -> Add10/1
  Demux2/1 -> Add25/1
  Constant17/1 -> Divide8/1
  Add26/1 -> Divide8/2
  Divide8/1 -> Product19/1
  Constant16/1 -> Add26/1
  Square/1 -> Add26/2
  Divide7/1 -> Square/1
  Gain10/1 -> Divide7/2
  Constant15/1 -> Divide7/1
  Product19/1 -> Switch4/1
  Constant14/1 -> Relational Operator/2
  Relational Operator/1 -> Switch4/2
  Constant10/1 -> Divide6/2
  Divide6/1 -> Relational Operator/1
  Gain9/1 -> Divide6/1
  [z] -> Gain9/1, Gain10/1
  Switch4/1 -> Switch2/1
  Switch2/1 -> Divide5/1  "ground"
  [Ena_ground] -> Switch2/2
  Demux2/2 -> Add11/1
  Demux3/1 -> Add25/2
  Demux3/2 -> Add11/2
  Demux3/3 -> Add10/2
  Gain8/1 -> Product18/2
  Gain7/1 -> Switch1/1
  Mux1/1 -> Gain7/1
  Constant13/1 -> Mux1/3
  Product18/1 -> Mux1/2
  Product17/1 -> Mux1/1
  [phidot] -> Product18/1
  [thetadot] -> Product17/1
  Switch1/1 -> Demux3/1  "gyro"
  Switch3/1 -> Demux2/1  "drag_torque"
  Product16/1 -> Switch3/1
  Mux/1 -> Product16/2
  [psidot] -> Mux/3
  [phidot] -> Mux/1
  [thetadot] -> Mux/2
  Gain6/1 -> Product16/1
  Constant12/1 -> Gain6/1
  Constant11/1 -> Switch1/3
  Constant9/1 -> Switch3/3
  [Ena_drag_torque] -> Switch3/2
  [Ena_gyro] -> Switch1/2
  Add25/1 -> Divide/1  "tau1"
  Add11/1 -> Divide1/1  "tau2"
  Add10/1 -> Divide2/1  "tau3"
  wind_power/1 -> Demux5/1
  Demux1/7 -> [Ena_wind]
  Demux1/6 -> [Ena_drag_torque]
  Demux1/5 -> [Ena_drag_force]
  Demux1/4 -> [Ena_ground]
  Demux1/3 -> [Ena_gyro]
  Demux1/1 -> [Ena_gravity]
  enables/1 -> Demux1/1
  [psidot0] -> Integrator2/2
  [thetadot0] -> Integrator1/2
  [phidot0] -> Integrator/2
  Demux/12 -> [psidot0]
  Demux/11 -> [thetadot0]
  Demux/10 -> [phidot0]
  Demux/9 -> [zdot0]
  Demux/8 -> [ydot0]
  Demux/7 -> [xdot0]
  Demux/6 -> [psi0]
  Demux/5 -> [theta0]
  Demux/4 -> [phi0]
  Demux/3 -> [z0]
  Demux/2 -> [y0]
  Demux/1 -> [x0]
  initial_value/1 -> Demux/1
  Divide5/1 -> Gain12/1, Scope1/1
  [z] -> z/1
  [phi] -> phi/1
  [theta] -> theta/1
  [psi] -> psi/1
  [xdot] -> xdot/1
  [ydot] -> ydot/1
  [zdot] -> zdot/1
  [phidot] -> phidot/1
  [thetadot] -> thetadot/1
  [psidot] -> psidot/1
  [y] -> y/1
  [x] -> x/1
  Constant6/1 -> Divide5/2
  F_thrust/1 -> Switch2/3, Switch4/3, Product19/2  "Fa"
  [thetadot] -> Product6/3
  [phidot] -> Product6/2
  [phidot] -> Product5/3
  [psidot] -> Product5/2
  [psidot] -> Product4/3
  [thetadot] -> Product4/2
  Add5/1 -> Integrator2/1
  Add4/1 -> Integrator1/1
  Add3/1 -> Integrator/1
  Constant5/1 -> Product6/1
  Constant4/1 -> Product5/1
  Constant3/1 -> Product4/1
  Product6/1 -> Add5/2
  Product5/1 -> Add4/2
  Product4/1 -> Add3/2
  Divide2/1 -> Add5/1
  Divide1/1 -> Add4/1
  Divide/1 -> Add3/1
  Constant2/1 -> Divide2/2
  Constant1/1 -> Divide1/2
  Constant/1 -> Divide/2
  M3/1 -> Product17/2, Gain8/1, Add10/3  "M3"
  M2/1 -> Add11/3  "M2"
  M1/1 -> Add25/3  "M1"
  Add/1 -> Integrator3/1
  u5/1 -> Add/1  "u5"
  Add1/1 -> Integrator9/1
  u6/1 -> Add1/1  "u6"
  Demux1/2 -> [Ena_euler_sat]
  Integrator8/1 -> Switch5/3  "phi_nolim"
  Integrator2/1 -> Integrator6/1, [psidot]  "psidot"
  Integrator1/1 -> [thetadot], Integrator5/1, Integrator7/1  "thetadot"
  Integrator/1 -> Integrator8/1, Integrator4/1, [phidot]  "phidot"
  [Ena_euler_sat] -> Switch/2
  [theta0] -> Integrator5/2
  Switch5/1 -> [phi]  "phi"
  Integrator4/1 -> Switch5/1  "phi_lim"
  [theta0] -> Integrator7/2
  Integrator7/1 -> Switch/3  "theta_nolim"
  Integrator5/1 -> Switch/1  "theta_lim"
  [psi0] -> Integrator6/2
  [phi0] -> Integrator8/2
  Switch/1 -> [theta]  "theta"
  Integrator6/1 -> [psi]  "psi"
  [Ena_euler_sat] -> Switch5/2
  [phi0] -> Integrator4/2

== matlab function uav_full_control/MATLAB Function4 ==
  data: x input; b output; y input; z input; phi input; theta input; psi input; xdot input; ydot input; zdot input; zeta input; xi input; p input; q input; r input
function b = b_function(x,y,z,phi,theta,psi,xdot,ydot,zdot,zeta,xi,p,q,r)

% prep
m=1.88;
g=9.81;
J1=1.453e-2;
J2=1.453e-2;
J3=2.884e-2;

input1=0;
input2=0;
input3=0;
input4=0;

sphi=sin(phi);
cphi=cos(phi);
stheta=sin(theta);
ctheta=cos(theta);
spsi=sin(psi);
cpsi=cos(psi);

% model dynamics
phi_dot=p+q*(sin(phi)*tan(theta))+r*(cos(phi)*tan(theta));
theta_dot=q*cos(phi)-r*sin(phi);
psi_dot=q*sin(phi)/cos(theta)+r*cos(phi)/cos(theta);


zeta_dot=xi;
xi_dot=input1;

p_dot=(J2-J3)/J1*q*r+1/J1*input2;
q_dot=(J3-J1)/J2*r*p+1/J2*input3;
r_dot=(J1-J2)/J3*p*q+1/J3*input4;

%others
phi_d_dot=p_dot+q_dot*sphi*tan(theta)+phi_dot*q*cphi*tan(theta)+theta_dot*q*sphi/(ctheta^2)+...
r_dot*cphi*tan(theta)-phi_dot*r*sphi*tan(theta)+theta_dot*r*cphi/(ctheta^2);

theta_d_dot=q_dot*cphi-phi_dot*q*sphi-r_dot*sphi-r*phi_dot*cphi;

psi_d_dot=q_dot*sphi/ctheta+q/(ctheta^2)*(phi_dot*cphi*ctheta+theta_dot*sphi*stheta)+...
r_dot*cphi/ctheta+r/(ctheta^2)*(-phi_dot*sphi*ctheta+theta_dot*cphi*stheta);

%%%--------------------------------------------------------------------------------------

%x

Cx=cphi*stheta*cpsi+sphi*spsi;

Cx_dot=-phi_dot*sphi*stheta*cpsi+theta_dot*cphi*ctheta*cpsi-psi_dot*cphi*stheta*spsi...
+phi_dot*cphi*spsi+psi_dot*sphi*cpsi;

Cx_d_dot=psi_d_dot*(-sphi*stheta*cpsi+cphi*spsi)+theta_d_dot*cphi*ctheta*cpsi...
+psi_d_dot*(-cphi*stheta*spsi+sphi*cpsi)-cphi*stheta*cpsi*(phi_dot^2+theta_dot^2+psi_dot^2)...
-2*phi_dot*theta_dot*sphi*ctheta*cpsi+2*phi_dot*psi_dot*sphi*stheta*spsi...
-2*theta_dot*psi_dot*cphi*ctheta*spsi-sphi*spsi*(phi_dot^2+psi_dot^2)+2*phi_dot*psi_dot*cphi*cpsi;

x_4dots=-1/m*(input1*Cx+2*xi*Cx_dot+zeta*Cx_d_dot); % Lf4h1(x)
LgLf3h1=-1/m*[Cx,...
    1/J1*zeta*(-sphi*stheta*cpsi+cphi*spsi),...
    1/J2*zeta*((-sphi*stheta*cpsi+cphi*spsi)*sphi*tan(theta)+cphi*ctheta*cpsi*cphi+...
    (-cphi*stheta*spsi+sphi*cpsi)*sphi/ctheta),...
    1/J3*zeta*((-sphi*stheta*cpsi+cphi*spsi)*cphi*tan(theta)-cphi*ctheta*cpsi*sphi+...
    (-cphi*stheta*spsi+sphi*cpsi)*cphi/ctheta)];

%y

Cy=cphi*stheta*spsi-sphi*cpsi;

Cy_dot=-phi_dot*sphi*stheta*spsi+theta_dot*cphi*ctheta*spsi+psi_dot*cphi*stheta*cpsi...
-phi_dot*cphi*cpsi+psi_dot*sphi*spsi;

Cy_d_dot=phi_d_dot*(-sphi*stheta*spsi-cphi*cpsi)+theta_d_dot*cphi*ctheta*spsi...
+psi_d_dot*(cphi*stheta*cpsi+sphi*spsi)-cphi*stheta*spsi*(phi_dot^2+theta_dot^2+psi_dot^2)...
-2*phi_dot*theta_dot*sphi*ctheta*spsi-2*phi_dot*psi_dot*sphi*stheta*cpsi...
+2*theta_dot*psi_dot*cphi*ctheta*cpsi+sphi*cpsi*(phi_dot^2+psi_dot^2)+2*phi_dot*psi_dot*cphi*spsi;

y_4dots=-1/m*(input1*Cy+2*xi*Cy_dot+zeta*Cy_d_dot);
LgLf3h2=-1/m*[Cy,...
    1/J1*zeta*(-sphi*stheta*spsi-cphi*cpsi),...
    1/J2*zeta*((-sphi*stheta*spsi-cphi*cpsi)*sphi*tan(theta)+cphi*ctheta*spsi*cphi+...
    (cphi*stheta*cpsi+sphi*spsi)*sphi/ctheta),...
    1/J3*zeta*((-sphi*stheta*spsi-cphi*cpsi)*cphi*tan(theta)-cphi*ctheta*spsi*sphi+...
    (cphi*stheta*cpsi+sphi*spsi)*cphi/ctheta)];
%z
Cz=cphi*ctheta;

Cz_dot=-phi_dot*sphi*ctheta-theta_dot*cphi*stheta;

Cz_d_dot=-phi_d_dot*sphi*ctheta-phi_dot^2*cphi*ctheta+2*phi_dot*theta_dot*sphi*stheta...
    -theta_d_dot*cphi*stheta-theta_dot^2*cphi*ctheta;

z_4dots=-1/m*(input1*Cz+2*xi*Cz_dot+zeta*Cz_d_dot);
LgLf3h3=-1/m*[Cz,...
    1/J1*zeta*(-sphi*ctheta),...
    1/J2*zeta*(-sphi*ctheta*sphi*tan(theta)-cphi*stheta*cphi),...
    1/J3*zeta*(-sphi*ctheta*cphi*tan(theta)+cphi*stheta*sphi)];

%psi

%psi_d_dot is defined above
LgLf1h4=[0,...
    0,...
    1/J2*sphi/ctheta,...
    1/J3*cphi/ctheta];
b=[x_4dots;y_4dots;z_4dots;psi_d_dot];
